simulink model "Simulink_21_ISFL"  (R2022b)
settings: Solver=VariableStepAuto  StartTime=0.0  StopTime=10.0  RelTol=1e-3
settings Model: Creator=a100142  LastModifiedBy=a100142

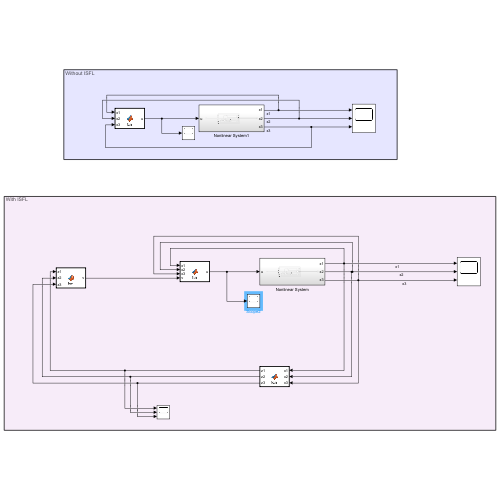
[thumbnail: Simulink's stored preview of the top-level diagram]
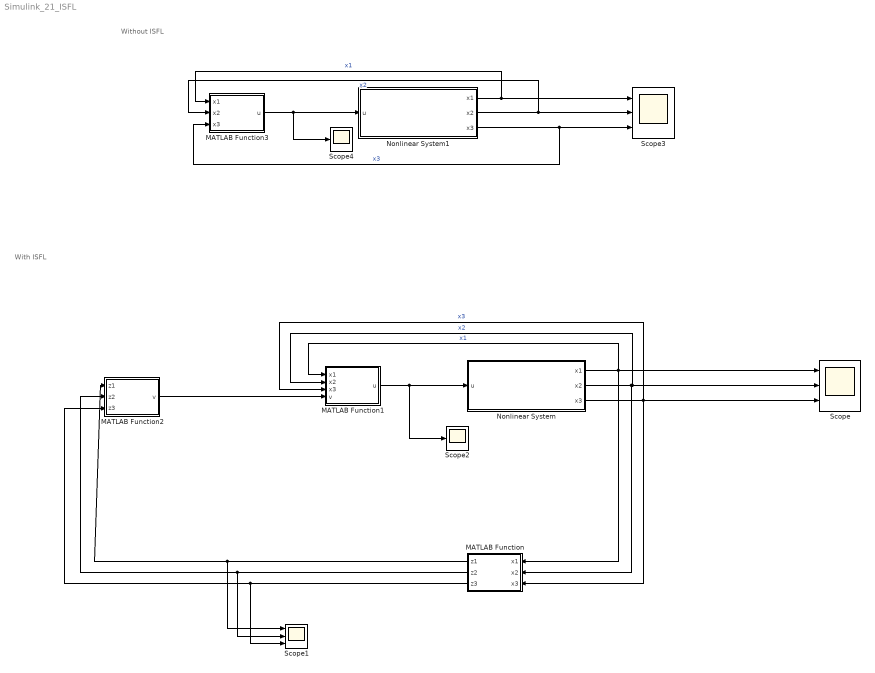
== system Simulink_21_ISFL ==
  note: With ISFL
  note: Without ISFL
  MATLAB Function : MATLAB Function  TreatAsAtomicUnit=on
  MATLAB Function1 : MATLAB Function  TreatAsAtomicUnit=on
  MATLAB Function2 : MATLAB Function  TreatAsAtomicUnit=on
  MATLAB Function3 : MATLAB Function  TreatAsAtomicUnit=on
  Nonlinear System : Subsystem
  Nonlinear System1 : Subsystem
  Scope : Scope  NumInputPorts=3
  Scope1 : Scope  NumInputPorts=3
  Scope2 : Scope
  Scope3 : Scope  NumInputPorts=3
  Scope4 : Scope
  wires:
  MATLAB Function1/1(u) -> Scope2/1, Nonlinear System/1(u)
  Nonlinear System/1(x1) -> MATLAB Function1/1(x1), MATLAB Function/1(x1), Scope/1  "x1"
  Nonlinear System/2(x2) -> MATLAB Function/2(x2), MATLAB Function1/2(x2), Scope/2  "x2"
  Nonlinear System/3(x3) -> MATLAB Function/3(x3), MATLAB Function1/3(x3), Scope/3  "x3"
  MATLAB Function2/1(v) -> MATLAB Function1/4(v)
  MATLAB Function/1(z1) -> Scope1/1, MATLAB Function2/1(z1)
  MATLAB Function/2(z2) -> Scope1/2, MATLAB Function2/2(z2)
  MATLAB Function/3(z3) -> Scope1/3, MATLAB Function2/3(z3)
  MATLAB Function3/1(u) -> Scope4/1, Nonlinear System1/1(u)
  Nonlinear System1/1(x1) -> MATLAB Function3/1(x1), Scope3/1  "x1"
  Nonlinear System1/2(x2) -> MATLAB Function3/2(x2), Scope3/2  "x2"
  Nonlinear System1/3(x3) -> MATLAB Function3/3(x3), Scope3/3  "x3"

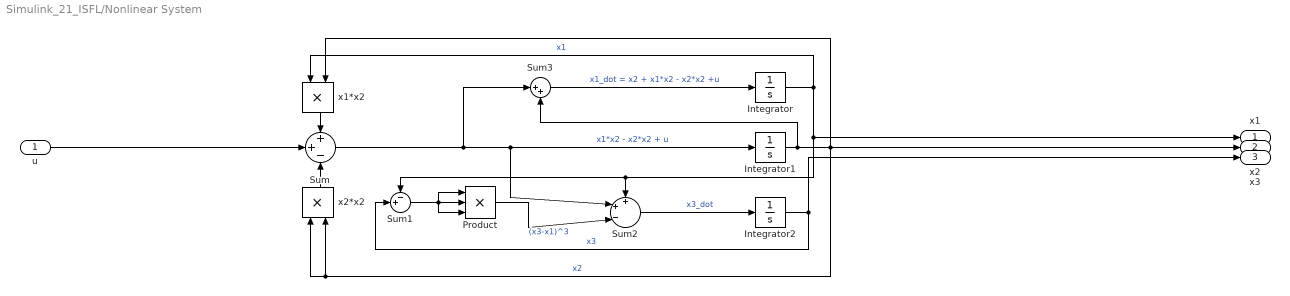
== system Simulink_21_ISFL/Nonlinear System ==
  u : Inport
  Integrator : Integrator  InitialCondition=1
  Integrator1 : Integrator  InitialCondition=1
  Integrator2 : Integrator  InitialCondition=1
  Product : Product  Inputs=3
  Sum : Sum  Inputs=++-
  Sum1 : Sum  Inputs=-+|
  Sum2 : Sum  Inputs=++-|
  Sum3 : Sum  Inputs=|++
  x1*x2 : Product
  x2*x2 : Product
  x1 : Outport
  x2 : Outport  Port=2
  x3 : Outport  Port=3
  wires:
  Sum3/1 -> Integrator/1  "x1_dot = x2 + x1*x2 - x2*x2 +u"
  Sum/1 -> Sum3/1, Integrator1/1, Sum2/2  "x1*x2 - x2*x2 + u"
  Product/1 -> Sum2/3  "(x3-x1)^3"
  Integrator/1 -> x1/1, Sum1/1, Sum2/1, x1*x2/1  "x1"
  Integrator1/1 -> x2/1, x2*x2/2, x2*x2/1, x1*x2/2, Sum3/2  "x2"
  x2*x2/1 -> Sum/3
  Integrator2/1 -> x3/1, Sum1/2  "x3"
  Sum1/1 -> Product/3, Product/2, Product/1
  x1*x2/1 -> Sum/1
  Sum2/1 -> Integrator2/1  "x3_dot"
  u/1 -> Sum/2

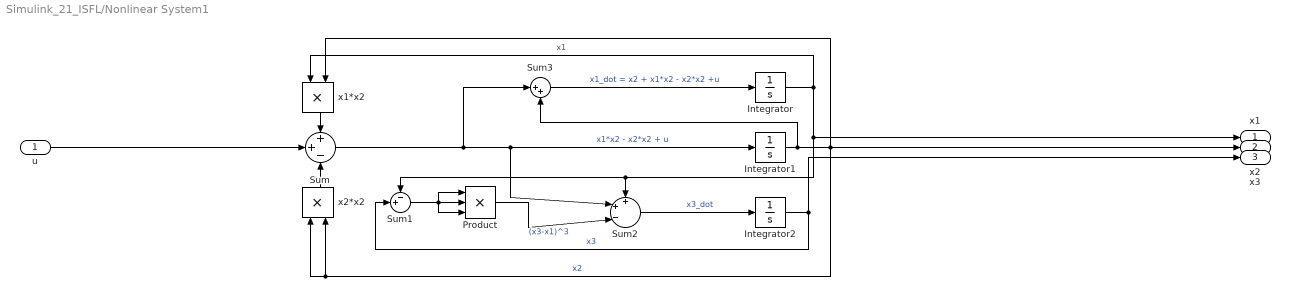
== system Simulink_21_ISFL/Nonlinear System1 ==
  u : Inport
  Integrator : Integrator  InitialCondition=1
  Integrator1 : Integrator  InitialCondition=1
  Integrator2 : Integrator  InitialCondition=1
  Product : Product  Inputs=3
  Sum : Sum  Inputs=++-
  Sum1 : Sum  Inputs=-+|
  Sum2 : Sum  Inputs=++-|
  Sum3 : Sum  Inputs=|++
  x1*x2 : Product
  x2*x2 : Product
  x1 : Outport
  x2 : Outport  Port=2
  x3 : Outport  Port=3
  wires:
  Sum3/1 -> Integrator/1  "x1_dot = x2 + x1*x2 - x2*x2 +u"
  Sum/1 -> Sum3/1, Integrator1/1, Sum2/2  "x1*x2 - x2*x2 + u"
  Product/1 -> Sum2/3  "(x3-x1)^3"
  Integrator/1 -> x1/1, Sum1/1, Sum2/1, x1*x2/1  "x1"
  Integrator1/1 -> x2/1, x2*x2/2, x2*x2/1, x1*x2/2, Sum3/2  "x2"
  x2*x2/1 -> Sum/3
  Integrator2/1 -> x3/1, Sum1/2  "x3"
  Sum1/1 -> Product/3, Product/2, Product/1
  x1*x2/1 -> Sum/1
  Sum2/1 -> Integrator2/1  "x3_dot"
  u/1 -> Sum/2

== matlab function Simulink_21_ISFL/MATLAB Function1 ==
  data: x1 input; x2 input; x3 input; v input; u output
function u= fcn(x1,x2,x3,v)

q = x1 - x3;
Lfq = x2 - x1 - (x1 - x3)^3;
Lf2q = x1*x2 - (3*(x1 - x3)^2 + 1)*(x2 + x1*x2 - x2^2) - x2^2 + 3*(x1 - x3)^2*(x1 + (x1 - x3)^3 + x1*x2 - x2^2);
Lf3q = (x2 + x1*x2 - x2^2)*(x2 - x2*(3*(x1 - x3)^2 + 1) + 3*(x1 - x3)^2*(x2 + 3*(x1 - x3)^2 + 1) - (6*x1 - 6*x3)*(x2 + x1*x2 - x2^2) + 3*(2*x1 - 2*x3)*(x1 + (x1 - x3)^3 + x1*x2 - x2^2)) - (9*(x1 - x3)^4 - (6*x1 - 6*x3)*(x2 + x1*x2 - x2^2) + 3*(2*x1 - 2*x3)*(x1 + (x1 - x3)^3 + x1*x2 - x2^2))*(x1 + (x1 - x3)^3 + x1*x2 - x2^2) + (- x2^2 + x1*x2)*(x1 - 2*x2 + 3*(x1 - 2*x2)*(x1 - x3)^2 - (3*(x1 - x3)^2 + 1)*(x1 - 2*x2 + 1));
LgLf2q = x1 - x2 - 9*(x1 - x3)^4 + 3*(x1 - 2*x2)*(x1 - x3)^2 - x2*(3*(x1 - x3)^2 + 1) + 3*(x1 - x3)^2*(x2 + 3*(x1 - x3)^2 + 1) - (3*(x1 - x3)^2 + 1)*(x1 - 2*x2 + 1);

Phi = [q; Lfq; Lf2q];

A = Lf3q;
B = LgLf2q;

% poles: -1, -2, -10

n1 = 20;
n2 = 32;
n3 = 13;

u =(v-A-n1*Phi(1)-n2*Phi(2)-n3*Phi(3))/B;

== matlab function Simulink_21_ISFL/MATLAB Function ==
  data: x1 input; z1 output; x2 input; x3 input; z2 output; z3 output
function [z1,z2,z3] = fcn(x1,x2,x3)

q = x1 -x3;
Lfq = x2 - x1 - (x1 - x3)^3;
Lf2q = x1*x2 - (3*(x1 - x3)^2 + 1)*(x2 + x1*x2 - x2^2) - x2^2 + 3*(x1 - x3)^2*(x1 + (x1 - x3)^3 + x1*x2 - x2^2);

z1 = q;
z2 = Lfq;
z3 = Lf2q;

== matlab function Simulink_21_ISFL/MATLAB Function2 ==
  data: z1 input; v output; z2 input; z3 input
function v = fcn(z1, z2, z3)

k1 = -1;
k2 = -1;
k3 = -1;

v = k1*z1+k2*z2+k3*z3;

== matlab function Simulink_21_ISFL/MATLAB Function3 ==
  data: x1 input; x2 input; x3 input; u output
function u= fcn(x1,x2,x3)

u = -1*x1-x2-x3;
